simulink model "PositionControlV2_1"  (Simulink 8.2)
settings: Solver=FixedStepDiscrete  StartTime=0.0  StopTime=Inf  RelTol=1e-3
PreLoadFcn:
  | Ts=0.001;
undefined symbols (not defined in the file): DiscIntNeverNeededParam
libraries: xpclib x5, speedgoatlib_IO102 x4, simulink x4, speedgoatlib_IO301 x4, xpcutilitieslib x3
settings Model: Creator=LukePH  LastModifiedBy=LukePH  SimulationMode=external  BufferReuse=off
settings DataIOCC: SignalLoggingSaveFormat=Dataset
settings OptimizationCC: BlockReduction=off  OptimizeBlockIOStorage=off  BufferReuse=off  ExpressionFolding=off  ExpressionDepthLimit=128  LocalBlockOutputs=off
settings DebuggingCC: FcnCallInpInsideContextMsg=EnableAllAsError  StateNameClashWarn=none
settings HardwareCC: ProdIntDivRoundTo=Zero  ProdEndianess=LittleEndian  ProdHWDeviceType=Generic->32-bit x86 compatible
settings RTWCC: SystemTargetFile=xpctarget.tlc  TemplateMakefile=xpc_default_tmf  Description=xPC Target  ProcessScript=xpctarget_make_rtw_hook  RTWCompilerOptimization=On
settings xpcTargetCC: TargetFcnLib=ansi_tfl_table_tmw.mat  CodeReplacementLibrary=XPC_BLAS  ParMdlRefBuildCompliant=on  ConcurrentExecutionCompliant=on  CombineSignalStateStructs=off  MATLABClassNameForMDSCustomization=xpcAperiodicCustomization  GRTInterface=on  GenerateAllocFcn=off  xPCTaskExecutionProfile=off  xPCRL32EventNumber=5000  xPCLoadParamSetFile=off  xPCConcurrentTasks=off  xPCEnableSFAnimation=off

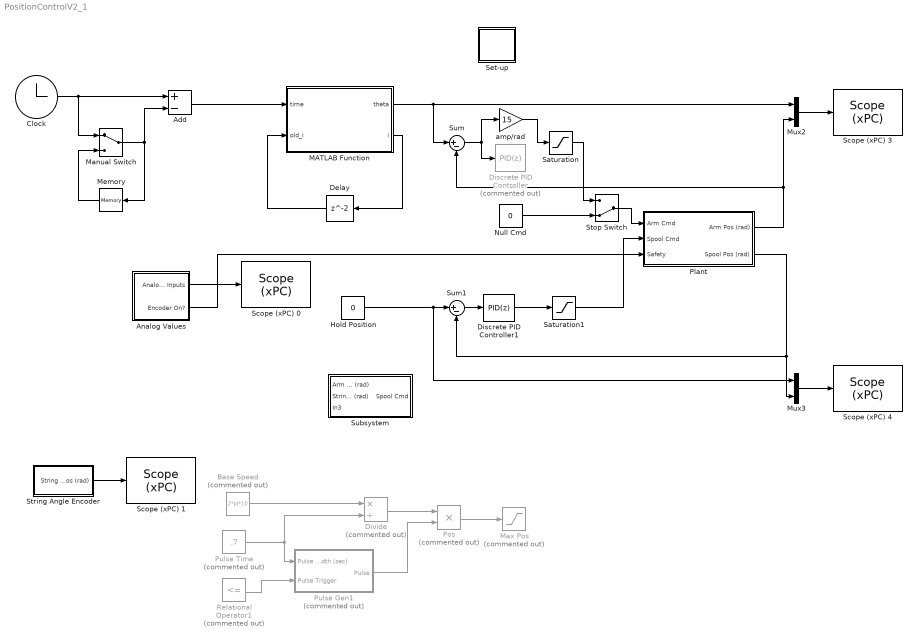
== system PositionControlV2_1 ==
  Add : Sum  Inputs=+-
  Analog Values : Subsystem
  Base Speed : Constant  Commented=on  Value=2*pi*10
  Clock : Clock
      settings: Decimation=5
  Delay : Delay  InitialCondition=1
  Discrete PID Controller : simulink/Continuous/PID Controller  Commented=on  Controller=PID  TimeDomain=Discrete-time  SampleTime=Ts  IntegratorMethod=Forward Euler  FilterMethod=Forward Euler  Form=Parallel  P=30  I=.15  D=1.5  N=100  InitialConditionSource=internal  InitialConditionForIntegrator=0  InitialConditionForFilter=0  ExternalReset=none  LimitOutput=on  UpperSaturationLimit=5  LowerSaturationLimit=-5  LinearizeAsGain=off  AntiWindupMode=clamping  Kb=1  TrackingMode=off  Kt=1  PParamMin=[]  PParamMax=[]  IParamMin=[]  IParamMax=[]  DParamMin=[]  DParamMax=[]  NParamMin=[]  NParamMax=[]  KbParamMin=[]  KbParamMax=[]  KtParamMin=[]  KtParamMax=[]  POutMin=[]  POutMax=[]  IOutMin=[]  IOutMax=[]  DOutMin=[]  DOutMax=[]  NOutMin=[]  NOutMax=[]  KbOutMin=[]  KbOutMax=[]  KtOutMin=[]  KtOutMax=[]  IntegratorOutMin=[]  IntegratorOutMax=[]  FilterOutMin=[]  FilterOutMax=[]  SumOutMin=[]  SumOutMax=[]  SumI1OutMin=[]  SumI1OutMax=[]  SumI2OutMin=[]  SumI2OutMax=[]  SumI3OutMin=[]  SumI3OutMax=[]  SumDOutMin=[]  SumDOutMax=[]  SaturationOutMin=[]  SaturationOutMax=[]  IntegratorContinuousStateAttributes=''  IntegratorStateMustResolveToSignalObject=off  IntegratorRTWStateStorageClass=Auto  FilterContinuousStateAttributes=''  FilterStateMustResolveToSignalObject=off  FilterRTWStateStorageClass=Auto
  Discrete PID Controller1 : simulink/Continuous/PID Controller  Controller=PID  TimeDomain=Discrete-time  SampleTime=Ts  IntegratorMethod=Forward Euler  FilterMethod=Forward Euler  Form=Parallel  P=4  I=.2  D=.25  N=100  InitialConditionSource=internal  InitialConditionForIntegrator=0  InitialConditionForFilter=0  ExternalReset=none  LimitOutput=on  UpperSaturationLimit=5  LowerSaturationLimit=-5  LinearizeAsGain=off  AntiWindupMode=clamping  Kb=1  TrackingMode=off  Kt=1  PParamMin=[]  PParamMax=[]  IParamMin=[]  IParamMax=[]  DParamMin=[]  DParamMax=[]  NParamMin=[]  NParamMax=[]  KbParamMin=[]  KbParamMax=[]  KtParamMin=[]  KtParamMax=[]  POutMin=[]  POutMax=[]  IOutMin=[]  IOutMax=[]  DOutMin=[]  DOutMax=[]  NOutMin=[]  NOutMax=[]  KbOutMin=[]  KbOutMax=[]  KtOutMin=[]  KtOutMax=[]  IntegratorOutMin=[]  IntegratorOutMax=[]  FilterOutMin=[]  FilterOutMax=[]  SumOutMin=[]  SumOutMax=[]  SumI1OutMin=[]  SumI1OutMax=[]  SumI2OutMin=[]  SumI2OutMax=[]  SumI3OutMin=[]  SumI3OutMax=[]  SumDOutMin=[]  SumDOutMax=[]  SaturationOutMin=[]  SaturationOutMax=[]  IntegratorContinuousStateAttributes=''  IntegratorStateMustResolveToSignalObject=off  IntegratorRTWStateStorageClass=Auto  FilterContinuousStateAttributes=''  FilterStateMustResolveToSignalObject=off  FilterRTWStateStorageClass=Auto
  Divide : Product  Commented=on  Inputs=*/
  Hold Position : Constant  Value=0
  MATLAB Function : MATLAB Function  TreatAsAtomicUnit=on
  Manual Switch : ManualSwitch
  Max Pos : Saturate  Commented=on  UpperLimit=2*pi*10  LowerLimit=-2*pi*10
  Memory : Memory  InheritSampleTime=on
  Mux2 : Mux  Inputs=2
  Mux3 : Mux  Inputs=2
  Null Cmd : Constant  Value=0
  Plant : Subsystem
  Pos : Product  Commented=on
  Pulse Gen1 : Subsystem  Commented=on
  Pulse Time : Constant  Commented=on  Value=.7
  Relational Operator1 : RelationalOperator  Commented=on  Operator=<=  OutDataTypeStr=boolean
  Saturation : Saturate  UpperLimit=5  LowerLimit=-5
  Saturation1 : Saturate  UpperLimit=3.5  LowerLimit=-3.5
  "Scope (xPC) 0 " : xpclib/Misc./Scope (xPC)   scopeno=1  scopetype=Target  autostart=on  viewmode=Numerical  formatstr='%15.6f'  grid=on  ylimits=[0,0]  nosamples=250  noprepostsamples=0  interleave=1  triggermode=FreeRun  triggersignal=1  trigsignalfromport=off  triggerlevel=0.0  triggerslope=Either  triggerscope=1  triggersample=0  filename=data.dat  mode=Lazy  writesize=512  autorestart=off  dynamicfilemode=off  maxwritefilesize=512*1024^2
  Scope (xPC) 1 : xpclib/Misc./Scope (xPC)   scopeno=2  scopetype=Target  autostart=on  viewmode=Graphical redraw  formatstr='%15.6f'  grid=on  ylimits=[-2*pi,2*pi]  nosamples=250  noprepostsamples=0  interleave=1  triggermode=FreeRun  triggersignal=1  trigsignalfromport=off  triggerlevel=0.0  triggerslope=Either  triggerscope=1  triggersample=0  filename=data.dat  mode=Lazy  writesize=512  autorestart=off  dynamicfilemode=off  maxwritefilesize=512*1024^2
  Scope (xPC) 3 : xpclib/Misc./Scope (xPC)   scopeno=3  scopetype=Target  autostart=on  viewmode=Graphical redraw  formatstr='%15.6f'  grid=on  ylimits=[-2*pi,2*pi]  nosamples=250  noprepostsamples=0  interleave=1  triggermode=FreeRun  triggersignal=1  trigsignalfromport=off  triggerlevel=0.0  triggerslope=Either  triggerscope=1  triggersample=0  filename=data.dat  mode=Lazy  writesize=512  autorestart=off  dynamicfilemode=off  maxwritefilesize=512*1024^2
  Scope (xPC) 4 : xpclib/Misc./Scope (xPC)   scopeno=4  scopetype=Target  autostart=on  viewmode=Graphical redraw  formatstr='%15.6f'  grid=on  ylimits=[-2*pi,2*pi]  nosamples=250  noprepostsamples=0  interleave=1  triggermode=FreeRun  triggersignal=1  trigsignalfromport=off  triggerlevel=0.0  triggerslope=Either  triggerscope=1  triggersample=0  filename=data.dat  mode=Lazy  writesize=512  autorestart=off  dynamicfilemode=off  maxwritefilesize=512*1024^2
  Set-up : Subsystem
  Stop Switch : ManualSwitch  CurrentSetting=0
  String Angle Encoder : Subsystem
  Subsystem : Subsystem
  Sum : Sum  Inputs=|+-
  Sum1 : Sum  Inputs=|+-
  amp/rad : Gain  Gain=15
  wires:
  Mux2/1 -> Scope (xPC) 3/1
  MATLAB Function/1(theta) -> Sum/1, Mux2/1
  Sum1/1 -> Discrete PID Controller1/1
  Discrete PID Controller1/1 -> Saturation1/1
  Mux3/1 -> Scope (xPC) 4/1
  Hold Position/1 -> Mux3/1, Sum1/1
  Delay/1 -> MATLAB Function/2(old_i)
  MATLAB Function/2(i) -> Delay/1
  Relational Operator1/1 -> Pulse Gen1/2(Pulse Trigger)
  Pulse Time/1 -> Pulse Gen1/1(Pulse Width (sec)), Divide/2
  Pulse Gen1/1(Pulse) -> Pos/2
  Pos/1 -> Max Pos/1
  Base Speed/1 -> Divide/1
  Divide/1 -> Pos/1
  Analog Values/1(Analog Inputs) -> "Scope (xPC) 0 "/1
  Plant/1(Arm Pos (rad)) -> Mux2/2, Sum/2
  Plant/2(Spool Pos (rad)) -> Sum1/2, Mux3/2
  Saturation1/1 -> Plant/2(Spool Cmd)
  Analog Values/2(Encoder On?) -> Plant/3(Safety)
  Clock/1 -> Add/1, Manual Switch/1
  Manual Switch/1 -> Memory/1, Add/2
  Memory/1 -> Manual Switch/2
  Add/1 -> MATLAB Function/1(time)
  Sum/1 -> amp/rad/1, Discrete PID Controller/1
  Null Cmd/1 -> Stop Switch/2
  Saturation/1 -> Stop Switch/1
  Stop Switch/1 -> Plant/1(Arm Cmd)
  amp/rad/1 -> Saturation/1
  String Angle Encoder/1(String Pos (rad)) -> Scope (xPC) 1/1

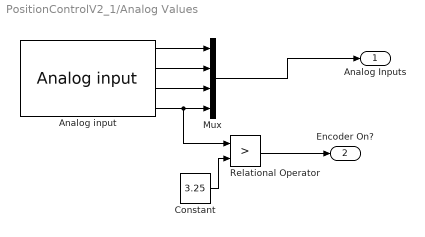
== system PositionControlV2_1/Analog Values ==
  Analog input : speedgoatlib_IO102/Analog input  id=1  channels=[1,2,3,4]  range=1  high_voltage=off  adCoupling=2  ts=Ts  pciSlot=-1
  Constant : Constant  Value=3.25
  Mux : Mux
  Relational Operator : RelationalOperator  Operator=>  OutDataTypeStr=fixdt(1,16)
  Analog Inputs : Outport
  Encoder On? : Outport  Port=2
  wires:
  Mux/1 -> Analog Inputs/1
  Relational Operator/1 -> Encoder On?/1
  Constant/1 -> Relational Operator/2
  Analog input/1 -> Mux/1
  Analog input/2 -> Mux/2
  Analog input/3 -> Mux/3
  Analog input/4 -> Relational Operator/1, Mux/4

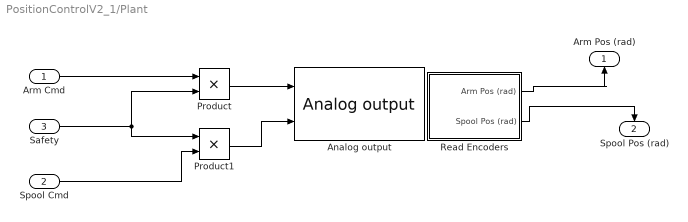
== system PositionControlV2_1/Plant ==
  Arm Cmd : Inport
  Spool Cmd : Inport  Port=2
  Safety : Inport  Port=3
  Analog output : speedgoatlib_IO102/Analog output  id=1  channels=[1,2]  range=1  ts=Ts  pciSlot=-1
  Product : Product
  Product1 : Product
  Read Encoders : Subsystem
  Arm Pos (rad) : Outport
  Spool Pos (rad) : Outport  Port=2
  wires:
  Read Encoders/2(Spool Pos (rad)) -> Spool Pos (rad)/1
  Spool Cmd/1 -> Product1/2
  Product1/1 -> Analog output/2
  Safety/1 -> Product1/1, Product/2
  Read Encoders/1(Arm Pos (rad)) -> Arm Pos (rad)/1
  Arm Cmd/1 -> Product/1
  Product/1 -> Analog output/1

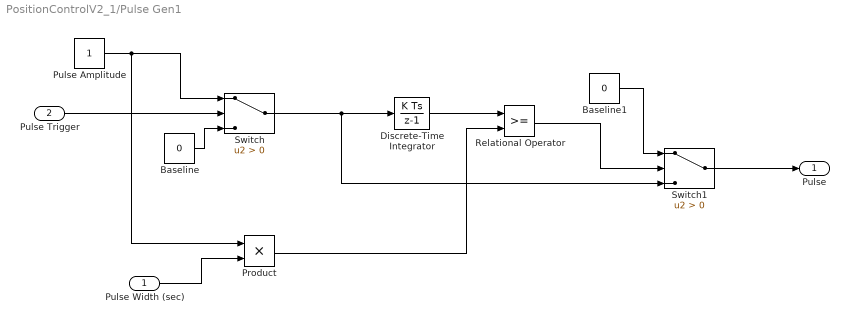
== system PositionControlV2_1/Pulse Gen1 ==
  Pulse Width (sec) : Inport
  Pulse Trigger : Inport  Port=2
  Baseline : Constant  Value=0
  Baseline1 : Constant  Value=0
  Discrete-Time Integrator : DiscreteIntegrator  SampleTime=Ts  ICPrevOutput=DiscIntNeverNeededParam  ICPrevScaledInput=DiscIntNeverNeededParam
  Product : Product
  Pulse Amplitude : Constant
  Relational Operator : RelationalOperator  OutDataTypeStr=boolean
  Switch : Switch  Criteria=u2 > Threshold
  Switch1 : Switch  Criteria=u2 > Threshold
  Pulse : Outport
  wires:
  Pulse Trigger/1 -> Switch/2
  Pulse Amplitude/1 -> Product/1, Switch/1
  Baseline/1 -> Switch/3
  Pulse Width (sec)/1 -> Product/2
  Switch/1 -> Switch1/3, Discrete-Time Integrator/1
  Product/1 -> Relational Operator/2
  Relational Operator/1 -> Switch1/2
  Baseline1/1 -> Switch1/1
  Switch1/1 -> Pulse/1
  Discrete-Time Integrator/1 -> Relational Operator/1

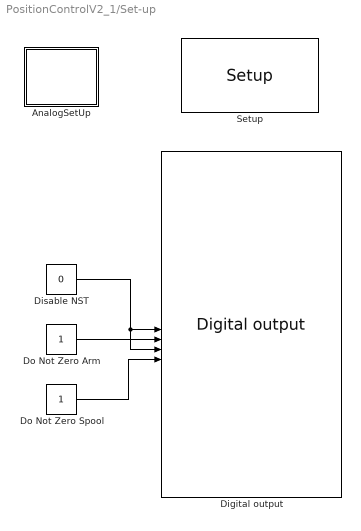
== system PositionControlV2_1/Set-up ==
  AnalogSetUp : Subsystem
  Digital output : speedgoatlib_IO301/DIO/Digital output  id=1  channelGroup=Lower  portType=32 ports of type double  lowerDirection=[0,0,0,0,0,0,1,1,1,1,1,1,1,1,1,1]  upperDirection=[1,1,1,1,1,1,1,1,0,0,0,0,0,0,0,0]  ts=Ts  pciSlot=-1
  Disable NST : Constant  Value=0
  Do Not Zero Arm : Constant
  Do Not Zero Spool : Constant
  Setup : speedgoatlib_IO301/Setup/Setup  group=Lower channel group setup  id=1  fpga1=speedgoat_IO301_CI_01230  pciSlot=-1  lowerDirection=[0,0,0,0,0,0,1,1,1,1,1,1,1,1,1,1]  lowerReset=[1]  lowerValue=[1]  upperDirection=[1, 1, 1, 1, 1, 1, 1, 1, 0, 0, 0, 0, 0, 0, 0, 0]  upperReset=[1]  upperValue=[0]
  wires:
  Disable NST/1 -> Digital output/19, Digital output/17
  Do Not Zero Arm/1 -> Digital output/18
  Do Not Zero Spool/1 -> Digital output/20

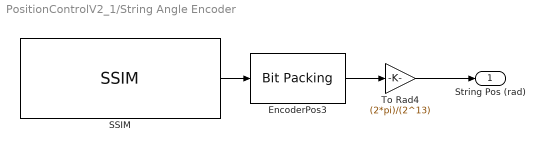
== system PositionControlV2_1/String Angle Encoder ==
  EncoderPos3 : xpcutilitieslib/Bit Packing   MaskBitPatterns={[0:12]}  MaskPackDataType=int32  MaskPackDataSize=[1]
  SSIM : speedgoatlib_IO301/SSI/SSIM  id=1  chan=[3]  coding=Binary  clockDivider=[200]  wordSize=[13]  TL=[0]  TP=[990]  ssiminv=off  ts=Ts  pciSlot=-1
  To Rad4 : Gain  Gain=(2*pi)/(2^13)  OutDataTypeStr=double
  String Pos (rad) : Outport
  wires:
  To Rad4/1 -> String Pos (rad)/1
  SSIM/1 -> EncoderPos3/1
  EncoderPos3/1 -> To Rad4/1

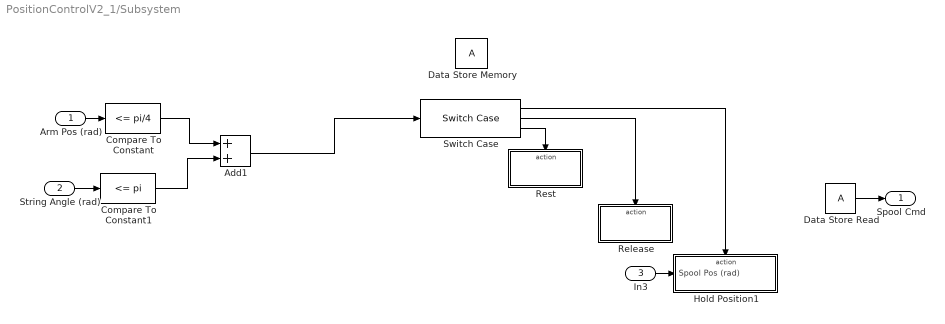
== system PositionControlV2_1/Subsystem ==
  Arm Pos (rad) : Inport
  String Angle (rad) : Inport  Port=2
  In3 : Inport  Port=3
  Add1 : Sum
  Compare To Constant : simulink/Logic and Bit Operations/Compare To Constant  relop=<=  const=pi/4  OutDataTypeStr=uint8
  Compare To Constant1 : simulink/Logic and Bit Operations/Compare To Constant  relop=<=  const=pi  OutDataTypeStr=uint8
  Data Store Memory : DataStoreMemory  ReadBeforeWriteMsg=warning  WriteAfterWriteMsg=warning  WriteAfterReadMsg=warning
  Data Store Read : DataStoreRead
  Hold Position1 : Subsystem  TreatAsAtomicUnit=on
  Release : Subsystem  TreatAsAtomicUnit=on
  Rest : Subsystem  TreatAsAtomicUnit=on
  Switch Case : SwitchCase  CaseConditions={[0,1],2}
  Spool Cmd : Outport
  wires:
  Compare To Constant/1 -> Add1/1
  Switch Case/2 -> Release/Action
  In3/1 -> Hold Position1/1(Spool Pos (rad))
  Switch Case/1 -> Hold Position1/Action
  Add1/1 -> Switch Case/1
  String Angle (rad)/1 -> Compare To Constant1/1
  Arm Pos (rad)/1 -> Compare To Constant/1
  Switch Case/3 -> Rest/Action
  Compare To Constant1/1 -> Add1/2
  Data Store Read/1 -> Spool Cmd/1

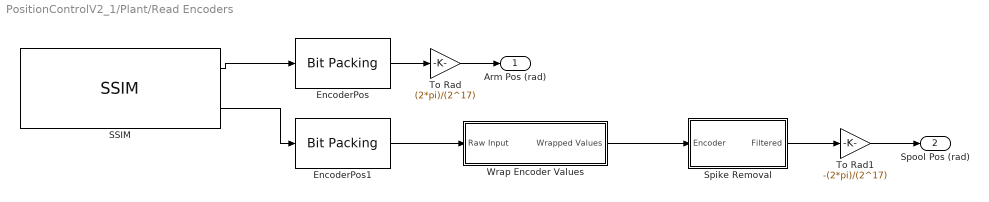
== system PositionControlV2_1/Plant/Read Encoders ==
  EncoderPos : xpcutilitieslib/Bit Packing   MaskBitPatterns={[0:16]}  MaskPackDataType=int32  MaskPackDataSize=[1]
  EncoderPos1 : xpcutilitieslib/Bit Packing   MaskBitPatterns={[0:16]}  MaskPackDataType=int32  MaskPackDataSize=[1]
  SSIM : speedgoatlib_IO301/SSI/SSIM  id=1  chan=[1:2]  coding=Gray  clockDivider=[200]  wordSize=[17]  TL=[0]  TP=[990]  ssiminv=off  ts=Ts  pciSlot=-1
  Spike Removal : Subsystem
  To Rad : Gain  Gain=(2*pi)/(2^17)  OutDataTypeStr=double
  To Rad1 : Gain  Gain=-(2*pi)/(2^17)  OutDataTypeStr=double
  Wrap Encoder Values : Subsystem
  Arm Pos (rad) : Outport
  Spool Pos (rad) : Outport  Port=2
  wires:
  SSIM/1 -> EncoderPos/1
  EncoderPos/1 -> To Rad/1
  To Rad/1 -> Arm Pos (rad)/1
  SSIM/2 -> EncoderPos1/1
  To Rad1/1 -> Spool Pos (rad)/1
  Spike Removal/1(Filtered) -> To Rad1/1
  EncoderPos1/1 -> Wrap Encoder Values/1(Raw Input)
  Wrap Encoder Values/1(Wrapped Values) -> Spike Removal/1(Encoder)

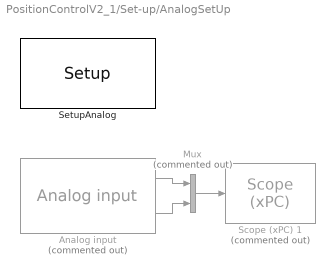
== system PositionControlV2_1/Set-up/AnalogSetUp ==
  Analog input : speedgoatlib_IO102/Analog input  Commented=on  id=1  channels=[1,2]  range=1  high_voltage=off  adCoupling=1  ts=Ts  pciSlot=-1
  Mux : Mux  Commented=on  Inputs=2
  Scope (xPC) 1 : xpclib/Misc./Scope (xPC)   Commented=on  scopeno=3  scopetype=Target  autostart=on  viewmode=Graphical redraw  formatstr='%15.6f'  grid=on  ylimits=[0,0]  nosamples=250  noprepostsamples=0  interleave=1  triggermode=FreeRun  triggersignal=1  trigsignalfromport=off  triggerlevel=0.0  triggerslope=Either  triggerscope=1  triggersample=0  filename=data.dat  mode=Lazy  writesize=512  autorestart=off  dynamicfilemode=off  maxwritefilesize=512*1024^2
  SetupAnalog : speedgoatlib_IO102/Setup  group=Analog input setup  id=1  range=+-10V  cal=off  pciSlot=-1  adChannelMode=Multiple-channel (enter number of channels below)  adChannel=4  adCoupling=Single-ended  daChannel=[1,2]  daReset=[1,1]  daInitValue=[0,0]  diChannel=[1]  doChannel=[1]  doReset=[1]  doInitValue=[0]
  wires:
  Mux/1 -> Scope (xPC) 1/1
  Analog input/1 -> Mux/1
  Analog input/2 -> Mux/2

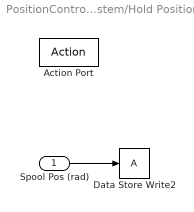
== system PositionControlV2_1/Subsystem/Hold Position1 ==
  Spool Pos (rad) : Inport
  Action Port : ActionPort
  Data Store Write2 : DataStoreWrite
  wires:
  Spool Pos (rad)/1 -> Data Store Write2/1

== system PositionControlV2_1/Subsystem/Release ==
  Action Port : ActionPort
  Data Store Write2 : DataStoreWrite
  Release Cmd : Constant
  wires:
  Release Cmd/1 -> Data Store Write2/1

== system PositionControlV2_1/Subsystem/Rest ==
  Action Port : ActionPort
  Constant : Constant  Value=0
  Data Store Write1 : DataStoreWrite
  wires:
  Constant/1 -> Data Store Write1/1

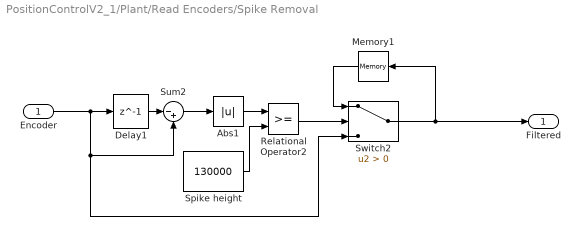
== system PositionControlV2_1/Plant/Read Encoders/Spike Removal ==
  Encoder : Inport
  Abs1 : Abs
  Delay1 : Delay  DelayLength=1  InitialCondition=0  SampleTime=Ts
  Memory1 : Memory  InheritSampleTime=on
  Relational Operator2 : RelationalOperator  OutDataTypeStr=boolean
  Spike height : Constant  Value=130000
  Sum2 : Sum  Inputs=|-+
  Switch2 : Switch  Criteria=u2 > Threshold  SampleTime=Ts
  Filtered : Outport
  wires:
  Switch2/1 -> Filtered/1, Memory1/1
  Delay1/1 -> Sum2/1
  Memory1/1 -> Switch2/1
  Encoder/1 -> Sum2/2, Switch2/3, Delay1/1
  Abs1/1 -> Relational Operator2/1
  Spike height/1 -> Relational Operator2/2
  Sum2/1 -> Abs1/1
  Relational Operator2/1 -> Switch2/2

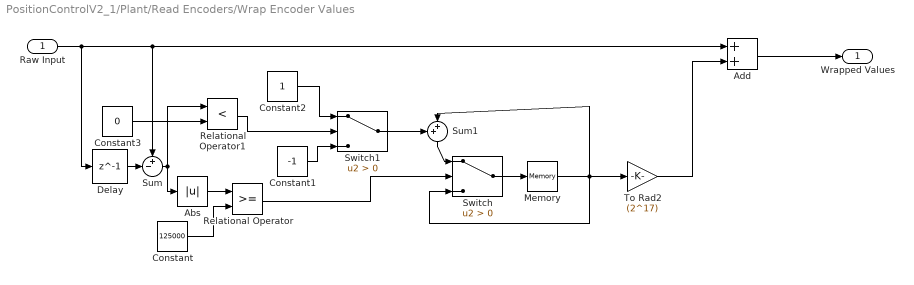
== system PositionControlV2_1/Plant/Read Encoders/Wrap Encoder Values ==
  Raw Input : Inport
  Abs : Abs
  Add : Sum
  Constant : Constant  Value=125000
  Constant1 : Constant  Value=-1
  Constant2 : Constant
  Constant3 : Constant  Value=0
  Delay : Delay  DelayLength=1  InitialCondition=0  SampleTime=Ts
  Memory : Memory  InheritSampleTime=on
  Relational Operator : RelationalOperator  OutDataTypeStr=boolean
  Relational Operator1 : RelationalOperator  Operator=<  OutDataTypeStr=boolean
  Sum : Sum  Inputs=+-|
  Sum1 : Sum  Inputs=++|
  Switch : Switch  Criteria=u2 > Threshold  SampleTime=Ts
  Switch1 : Switch  Criteria=u2 > Threshold  SampleTime=Ts
  To Rad2 : Gain  Gain=(2^17)  OutDataTypeStr=double
  Wrapped Values : Outport
  wires:
  Raw Input/1 -> Delay/1, Sum/1, Add/1
  Add/1 -> Wrapped Values/1
  Constant/1 -> Relational Operator/2
  Relational Operator/1 -> Switch/2
  Sum1/1 -> Switch/1
  Delay/1 -> Sum/2
  Switch/1 -> Memory/1
  Memory/1 -> Sum1/2, Switch/3, To Rad2/1
  Switch1/1 -> Sum1/1
  Constant1/1 -> Switch1/3
  Relational Operator1/1 -> Switch1/2
  Constant2/1 -> Switch1/1
  Sum/1 -> Relational Operator1/1, Abs/1
  Abs/1 -> Relational Operator/1
  Constant3/1 -> Relational Operator1/2
  To Rad2/1 -> Add/2

== matlab function MATLAB Function ==
  data: time input double; theta output double; old_i input double; i output double
function [theta, i] = TrajectoryTimeMap(time,old_i)
%#codegen
% Timing Points
T = [.75, 1.025, 1.125, 1.25, 3.25];

Pts = [[0,    pi,        0];...
       [T(1), pi+1.25,   0];...
       [T(2), pi,      -.25*pi/(T(3)-T(2))];... % Linear regime
       [T(3), pi-pi/4,   -.25*pi/(T(3)-T(2))];... % Linear regime
       [T(4), pi-1.125,    0];...
       [T(5), pi-1.125,    0]];
  
% Generate Path
[t, Th] = SplinePath(Pts,100);
accu = 10^6;        % Accuracy

% Check to see if end of simulation
if time > max(T)
    theta = Th(end);
    i = old_i;
else
    % Find closest time
    [Val, I] = min(round(accu*abs(t - time))/accu);
    theta = Th(I);
    i = I;
end %If
end % Function


%%%%%%%%%%%%%%%%%%%%%%%%%%%%%%%%%%%%%%%%%%%%%%%%%%%%%%%%%%%%%%%%%%%%%%%%%%
function [ t, X ] = SplinePath( Points, n )
% Create Path, fits curve between Points (t,x dx) every n timestep

t = linspace(Points(1,1), Points(end,1),n); 
dt = t(2) - t(1);
X = zeros(1,n);
X(1)    = Points(1,2);

for i=2:n
   k = find(Points(:,1)>=t(i));
   m = k(1);
   x1 = Points(m-1,1);
   x2 = Points(m,1);
   y1 = Points(m-1,2);
   y2 = Points(m,2);
   k1 = Points(m-1,3);
   k2 = Points(m,3);
   
   g = ( t(i) - x1 )/( x2 - x1 );
   a = k1*(x2-x1)-(y2-y1);
   b =-k2*(x2-x1)+(y2-y1);
   
   X(i) = (1-g)*y1 + g*y2 +g*(1-g)*(a*(1-g)+b*g);
end

end% SplinePathFunction
